simulink model "fzhomework"  (R2019a)
settings: Solver=VariableStepAuto  StartTime=0.0  StopTime=10.0  RelTol=1e-3
settings Model: Creator=Administrator  LastModifiedBy=Administrator

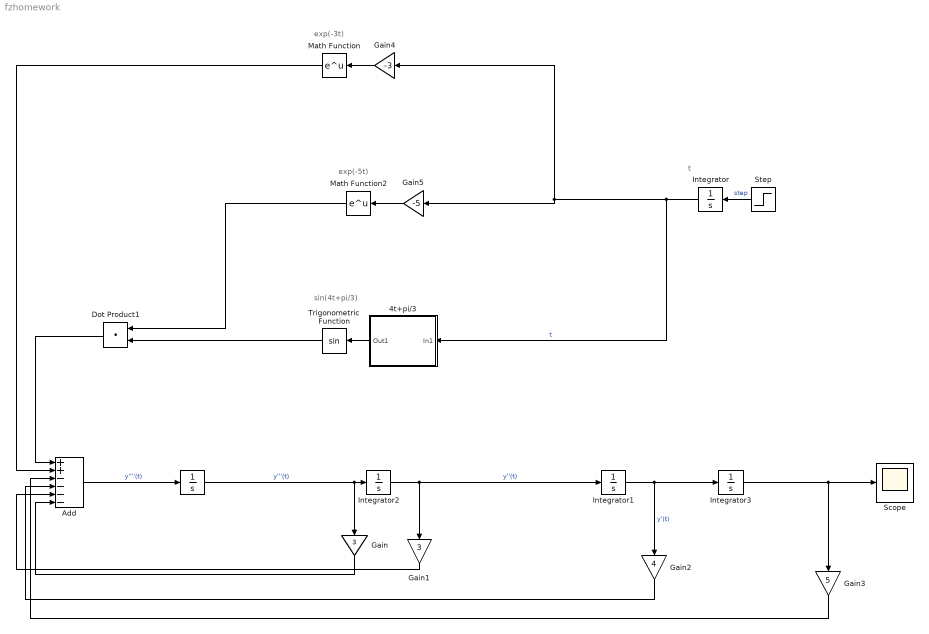
== system fzhomework ==
  note: t
  note: sin(4t+pi/3)
  note: exp(-5t)
  note: exp(-3t)
  " " : Integrator  InitialCondition=0.2
  4t+pi/3 : Subsystem
  Add : Sum  Inputs=++----
  Dot Product1 : DotProduct  InputSameDT=on  OutDataTypeStr=Inherit: Inherit via internal rule
  Gain : Gain  Gain=3
  Gain1 : Gain  Gain=3
  Gain2 : Gain  Gain=4
  Gain3 : Gain  Gain=5
  Gain4 : Gain  Gain=-3
  Gain5 : Gain  Gain=-5
  Integrator : Integrator
  Integrator1 : Integrator  InitialCondition=0.5
  Integrator2 : Integrator  InitialCondition=0.5
  Integrator3 : Integrator  InitialCondition=1
  Math Function : Math  SaturateOnIntegerOverflow=on
  Math Function2 : Math  SaturateOnIntegerOverflow=on
  Scope : Scope
  Step : Step  SampleTime=0
  Trigonometric Function : Trigonometry
  wires:
  Add/1 -> " "/1  "y''''(t)"
  " "/1 -> Gain/1, Integrator2/1  "y'''(t)"
  Integrator2/1 -> Gain1/1, Integrator1/1  "y''(t)"
  Integrator1/1 -> Integrator3/1, Gain2/1  "y'(t)"
  Gain/1 -> Add/6
  Gain1/1 -> Add/5
  Gain2/1 -> Add/4
  Integrator3/1 -> Gain3/1, Scope/1
  Gain3/1 -> Add/3
  Dot Product1/1 -> Add/1
  Math Function/1 -> Add/2
  Trigonometric Function/1 -> Dot Product1/2
  Math Function2/1 -> Dot Product1/1
  Gain4/1 -> Math Function/1
  Gain5/1 -> Math Function2/1
  4t+pi/3/1(Out1) -> Trigonometric Function/1
  Integrator/1 -> Gain4/1, Gain5/1, 4t+pi/3/1(In1)  "t"
  Step/1 -> Integrator/1  "step"

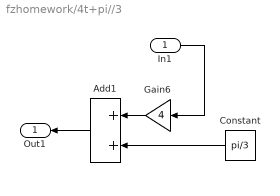
== system fzhomework/4t+pi//3 ==
  In1 : Inport
  Add1 : Sum
  Constant : Constant  Value=pi/3
  Gain6 : Gain  Gain=4
  Out1 : Outport
  wires:
  Constant/1 -> Add1/2
  Gain6/1 -> Add1/1
  Add1/1 -> Out1/1
  In1/1 -> Gain6/1
